simulink model "FOC_LSM"  (R2026a)
settings: Solver=VariableStepAuto  StopTime=5  MaxStep=0.001
values from neighbouring files (symbols this model uses):
  airgap_vec = 14.5:1:16.5    [CargarDatosModeloLSM.m]
  force_drag_vec = []    [CargarDatosModeloLSM.m]
  hems_n = 4    [CargarDatosModeloLSM.m]
  kd = 0.0518    [CargarDatosModeloLSM.m]
  mass = 250    [CargarDatosModeloLSM.m]
  max_current = 100    [CargarDatosModeloLSM.m]
  max_voltage = 300    [CargarDatosModeloLSM.m]
  real_airgap = 14.5    [CargarDatosModeloLSM.m]
  speed_drag_vec = 0:5:60    [CargarDatosModeloLSM.m]
undefined symbols (not defined in the file or in its folder): angulos, frac_polar, fuerza, magnitude, Resistencia
libraries: slpidlib x3
settings Model: Creator=USUARIO  LastModifiedBy=osganig
settings SolverCC: InitialStep=0.000001
settings SimscapeCC: SimscapeNominalValues="[{\"value\":\"1\",\"unit\":\"A\"},{\"value\":\"1\",\"unit\":\"bar\"},{\"value\":\"1\",\"unit\":\"cm^2\"},{\"value\":\"1\",\"unit\":\"cm^3/s\"},{\"value\":\"1\",\"unit\":\"kJ/kg\"},{\"value\":\"1\",\"unit\":\"kW\"},{\"value\":\"1\",\"unit\":\"l\"},{\"value\":\"1\",\"unit\":\"N\"},{\"value\":\"1\",\"unit\":\"N*m\"},{\"value\":\"1\",\"unit\":\"V\"}]"  SimscapeLogType=none  SimscapeLogDataHistory=5000.0

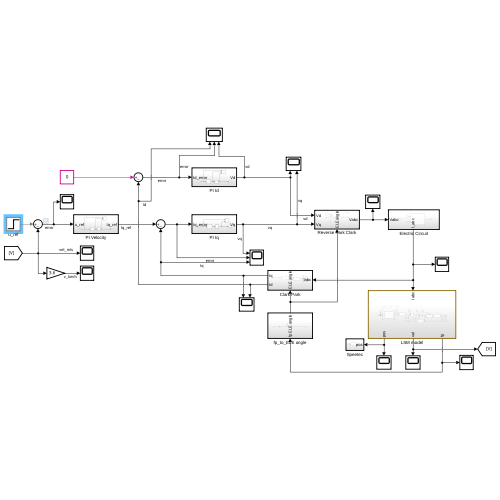
[thumbnail: Simulink's stored preview of the top-level diagram]
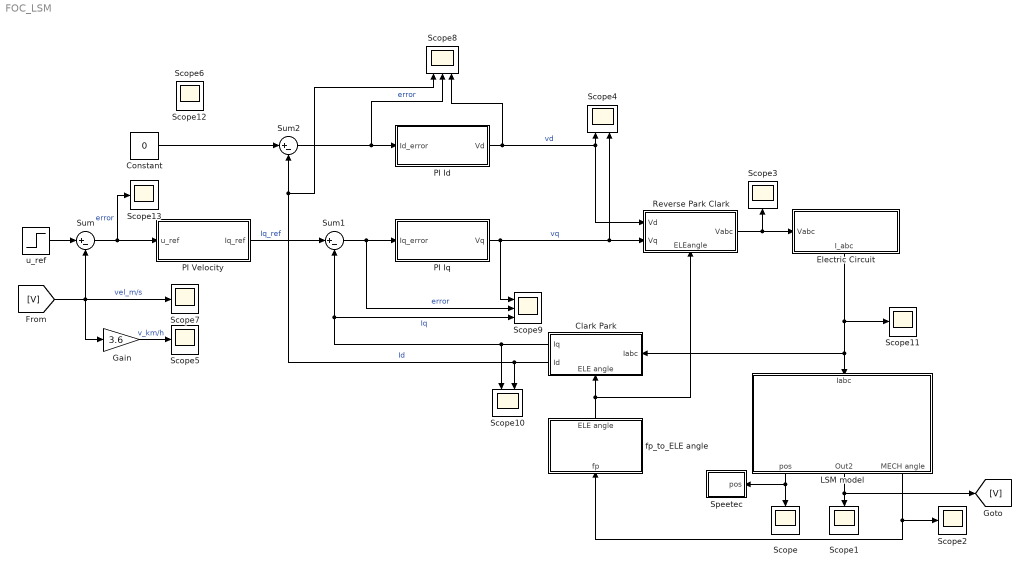
== system FOC_LSM ==
  Clark Park : Subsystem
      settings: PortSchema="{\"entries\":[{\"content\":{\"sides\":[{\"content\":{\"connectorIds\":[\"Out1\",\"Out2\"]},\"type\":\"ConnectorPlacement.EquallySpacedRectSide\",\"uuid\":\"b73a0972-bf68-45ae-9239-d3343df02446\"},{\"content\":{\"connectorIds\":[\"In2\"],\"side\":\"RIGHT\"},\"type\":\"ConnectorPlacement.EquallySpacedRectSide\",\"uuid\":\"fec89271-c2ef-4885-992a-4c0db260d6e2\"},{\"content\":{\"side\":\"TOP\"},\"type\":\"ConnectorPlacement.EquallySpacedRectSide\",\"uuid\":\"51dbb3d3-34a9-43d7-9c98-9fa2f2011719\"},{\"content\":{\"connectorIds\":[\"In1\"],\"side\":\"BOTTOM\"},\"type\":\"ConnectorPlacement.EquallySpacedRectSide\",\"uuid\":\"eab6f42e-44ed-4b27-921c-43f03788cacc\"}]},\"type\":\"ConnectorPlacement.EquallySpacedConnector\",\"uuid\":\"a64495c7-a005-4dee-b109-5230f9247adc\"}],\"packageUris\":[\"http://schema.mathworks.com/mf0/Connector/R2020b\"],\"version\":\"1.0\"}"
  Constant : Constant  Value=0
  Electric Circuit : Subsystem
      settings: PortSchema="{\"entries\":[{\"content\":{\"sides\":[{\"content\":{\"connectorIds\":[\"In1\"]},\"type\":\"ConnectorPlacement.EquallySpacedRectSide\",\"uuid\":\"3f81a6db-fb69-453a-a09a-736cf4e6fbdf\"},{\"content\":{\"side\":\"RIGHT\"},\"type\":\"ConnectorPlacement.EquallySpacedRectSide\",\"uuid\":\"28f19065-0fce-4caf-9d5e-808d35e6acc4\"},{\"content\":{\"side\":\"TOP\"},\"type\":\"ConnectorPlacement.EquallySpacedRectSide\",\"uuid\":\"0f0f3d94-64b2-4ad8-85c5-3a76de2037a2\"},{\"content\":{\"connectorIds\":[\"Out1\"],\"side\":\"BOTTOM\"},\"type\":\"ConnectorPlacement.EquallySpacedRectSide\",\"uuid\":\"1e961944-9c4a-4342-972a-1097eb822071\"}]},\"type\":\"ConnectorPlacement.EquallySpacedConnector\",\"uuid\":\"ca84a14e-6f4b-4b2e-8a9f-b6683e76143b\"}],\"packageUris\":[\"http://schema.mathworks.com/mf0/Connector/R2020b\"],\"version\":\"1.0\"}"
  Gain : Gain  Gain=3.6
  LSM model : Subsystem
      settings: PortSchema="{\"entries\":[{\"content\":{\"sides\":[{\"content\":{},\"type\":\"ConnectorPlacement.EquallySpacedRectSide\",\"uuid\":\"cac53d69-c428-44dc-bdf5-c688872b0596\"},{\"content\":{\"side\":\"RIGHT\"},\"type\":\"ConnectorPlacement.EquallySpacedRectSide\",\"uuid\":\"eab58244-5d35-448a-9540-885c93543b87\"},{\"content\":{\"connectorIds\":[\"In1\"],\"side\":\"TOP\"},\"type\":\"ConnectorPlacement.EquallySpacedRectSide\",\"uuid\":\"c64ce138-6960-4dd5-9e90-e1ffecc69b70\"},{\"content\":{\"connectorIds\":[\"Out1\",\"Out2\",\"Out3\"],\"side\":\"BOTTOM\"},\"type\":\"ConnectorPlacement.EquallySpacedRectSide\",\"uuid\":\"eda83129-b662-4da7-9603-68b1882420cc\"}]},\"type\":\"ConnectorPlacement.EquallySpacedConnector\",\"uuid\":\"82b650b8-86c6-4f03-ba07-634d14e4b94d\"}],\"packageUris\":[\"http://schema.mathworks.com/mf0/Connector/R2020b\"],\"version\":\"1.0\"}"
  PI Id : Subsystem
  PI Iq : Subsystem
  PI Velocity : Subsystem
  Reverse Park Clark : Subsystem
      settings: PortSchema="{\"entries\":[{\"content\":{\"sides\":[{\"content\":{\"connectorIds\":[\"In1\",\"In2\"]},\"type\":\"ConnectorPlacement.EquallySpacedRectSide\",\"uuid\":\"bb4b1d20-48ba-4b2f-b253-a250226ab501\"},{\"content\":{\"connectorIds\":[\"Out1\"],\"side\":\"RIGHT\"},\"type\":\"ConnectorPlacement.EquallySpacedRectSide\",\"uuid\":\"4768cfae-b67e-4820-9de3-2f5fe637e53a\"},{\"content\":{\"side\":\"TOP\"},\"type\":\"ConnectorPlacement.EquallySpacedRectSide\",\"uuid\":\"af639b0a-05db-45f8-bbbc-8f88455894ca\"},{\"content\":{\"connectorIds\":[\"In3\"],\"side\":\"BOTTOM\"},\"type\":\"ConnectorPlacement.EquallySpacedRectSide\",\"uuid\":\"149993ad-8fc7-43c9-baef-e4c40b0fb2ea\"}]},\"type\":\"ConnectorPlacement.EquallySpacedConnector\",\"uuid\":\"6dc62ad4-a38d-4494-a0f6-179f186f788d\"}],\"packageUris\":[\"http://schema.mathworks.com/mf0/Connector/R2020b\"],\"version\":\"1.0\"}"
  Scope{,1..3,5..7,11..13} (10 alike) : Scope
      Scope settings: ActiveDisplayYMinimum=-44.742643524791177  ActiveDisplayYMaximum=63.649983628393485
      Scope1 settings: ActiveDisplayYMinimum=-1  ActiveDisplayYMaximum=1  DataLoggingVariableName=ScopeData2
      Scope11 settings: ActiveDisplayYMinimum=-239.32432239172496  ActiveDisplayYMaximum=188.83608076645984  DataLoggingVariableName=ScopeData8
      Scope13 settings: ActiveDisplayYMinimum=-4.7371182514863284  ActiveDisplayYMaximum=8.95741762391783  DataLoggingVariableName=ScopeData26
      Scope2 settings: ActiveDisplayYMinimum=-0.25  ActiveDisplayYMaximum=2.25  DataLoggingVariableName=ScopeData3
      Scope3 settings: ActiveDisplayYMinimum=-282.3019987095613  ActiveDisplayYMaximum=236.76374680543654  DataLoggingVariableName=ScopeData7
      Scope5 settings: ActiveDisplayYMinimum=-77.099854779742387  ActiveDisplayYMaximum=22.66504143319689  DataLoggingVariableName=ScopeData22
      Scope7 settings: ActiveDisplayYMinimum=4.6850634488954057  ActiveDisplayYMaximum=8.1784524143386932  DataLoggingVariableName=ScopeData17
      Scope12 settings: DataLoggingVariableName=ScopeData24
      Scope6 settings: ActiveDisplayYMinimum=-26.658365067541684  ActiveDisplayYMaximum=23.617816668325265  DataLoggingVariableName=ScopeData23
  Scope10 : Scope  NumInputPorts=2
      settings: ActiveDisplayYMinimum=-159.849934056899  ActiveDisplayYMaximum=156.59274633785697  DataLoggingVariableName=ScopeData21
  Scope4 : Scope  NumInputPorts=2
      settings: ActiveDisplayYMinimum=-644.81411467829275  ActiveDisplayYMaximum=391.29333465512445  DataLoggingVariableName=ScopeData9
  Scope8 : Scope  NumInputPorts=3
      settings: ActiveDisplayYMinimum=-641.93741582792154  ActiveDisplayYMaximum=154.89056521574875  DataLoggingVariableName=ScopeData18
  Scope9 : Scope  NumInputPorts=3
      settings: ActiveDisplayYMinimum=-2.3010895783885954  ActiveDisplayYMaximum=2.3440027579560128  DataLoggingVariableName=ScopeData19
  Speetec : Subsystem
  Sum : Sum  Inputs=|+-
  Sum1 : Sum  Inputs=|+-
  Sum2 : Sum  Inputs=|+-
  fp_to_ELE angle : Subsystem
      settings: PortSchema="{\"entries\":[{\"content\":{\"sides\":[{\"content\":{},\"type\":\"ConnectorPlacement.EquallySpacedRectSide\",\"uuid\":\"b73a0972-bf68-45ae-9239-d3343df02446\"},{\"content\":{\"side\":\"RIGHT\"},\"type\":\"ConnectorPlacement.EquallySpacedRectSide\",\"uuid\":\"fec89271-c2ef-4885-992a-4c0db260d6e2\"},{\"content\":{\"connectorIds\":[\"Out1\"],\"side\":\"TOP\"},\"type\":\"ConnectorPlacement.EquallySpacedRectSide\",\"uuid\":\"51dbb3d3-34a9-43d7-9c98-9fa2f2011719\"},{\"content\":{\"connectorIds\":[\"In1\"],\"side\":\"BOTTOM\"},\"type\":\"ConnectorPlacement.EquallySpacedRectSide\",\"uuid\":\"4816d69c-9e54-4057-b439-390caef350ee\"}]},\"type\":\"ConnectorPlacement.EquallySpacedConnector\",\"uuid\":\"a64495c7-a005-4dee-b109-5230f9247adc\"}],\"packageUris\":[\"http://schema.mathworks.com/mf0/Connector/R2020b\"],\"version\":\"1.0\"}"
  u_ref : Step  FinalValue=speed_reference_ms  SampleTime=0
  wires:
  Constant/1 -> Sum2/1
  LSM model/3(MECH angle) -> fp_to_ELE angle/1(fp), Scope2/1
  Clark Park/2(Id) -> Scope10/2, Scope8/1, Sum2/2  "Id"
  fp_to_ELE angle/1(ELE angle) -> Reverse Park Clark/3(ELEangle), Clark Park/1(ELE angle)
  Clark Park/1(Iq) -> Scope10/1, Scope9/3, Sum1/2  "Iq"
  Electric Circuit/1(I_abc) -> LSM model/1(Iabc), Clark Park/2(Iabc), Scope11/1
  u_ref/1 -> Sum/1
  Sum1/1 -> PI Iq/1(Iq_error), Scope9/2  "error"
  LSM model/1(pos) -> Scope/1, Speetec/1(pos)
  LSM model/2(Out2) -> Scope1/1, [V]
  PI Id/1(Vd) -> Scope8/3, Reverse Park Clark/1(Vd), Scope4/1  "vd"
  [V] -> Scope7/1, Gain/1, Sum/2  "vel_m/s"
  Sum/1 -> Scope13/1, PI Velocity/1(u_ref)  "error"
  Sum2/1 -> PI Id/1(Id_error), Scope8/2  "error"
  PI Iq/1(Vq) -> Reverse Park Clark/2(Vq), Scope4/2, Scope9/1  "vq"
  Reverse Park Clark/1(Vabc) -> Electric Circuit/1(Vabc), Scope3/1
  PI Velocity/1(Iq_ref) -> Sum1/1  "Iq_ref"
  Gain/1 -> Scope5/1  "v_km/h"

== system FOC_LSM/Clark Park ==
  ELE angle : Inport
  Iabc : Inport  Port=2
  Clarke Transform : MATLAB Function  TreatAsAtomicUnit=on
  Clarke to Park Angle Transform : MATLAB Function  TreatAsAtomicUnit=on
  Demux : Demux  Outputs=3
  Terminator : Terminator
  Iq : Outport
  Id : Outport  Port=2
  wires:
  Iabc/1 -> Clarke Transform/1(abc)
  ELE angle/1 -> Clarke to Park Angle Transform/2(ELE_angle)
  Clarke to Park Angle Transform/1(dq0) -> Demux/1
  Demux/1 -> Id/1
  Demux/2 -> Iq/1
  Demux/3 -> Terminator/1
  Clarke Transform/1(AlphaBeta0) -> Clarke to Park Angle Transform/1(AlphaBeta0)

== system FOC_LSM/Electric Circuit ==
  Vabc : Inport
  Constant : Constant  Value=0.01
  Equivalente eléctrico : Subsystem
  I_abc : Outport
  wires:
  Equivalente eléctrico/1(I UVW) -> I_abc/1
  [V_abc] -> Equivalente eléctrico/2(Voltaje)
  Constant/1 -> Equivalente eléctrico/1(Inductancia)
  Vabc/1 -> [V_abc]

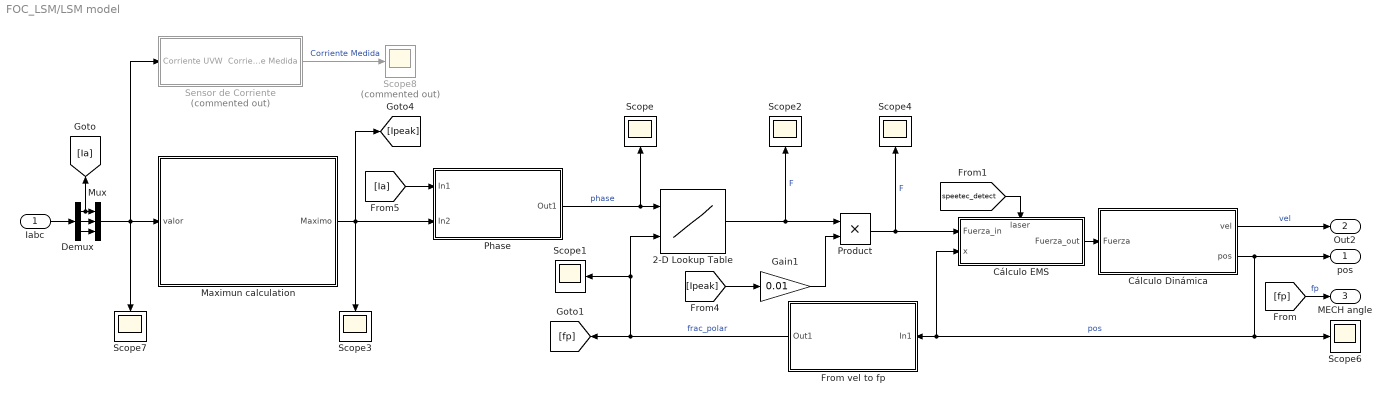
== system FOC_LSM/LSM model ==
  Iabc : Inport
  2-D Lookup Table : Lookup_n-D  BreakpointsForDimension1=angulos  BreakpointsForDimension2=frac_polar  Table=fuerza  InternalRulePriority=Speed  RndMeth=Simplest
      settings: InputPortMap=u0,u1
  Cálculo Dinámica : Subsystem
  Cálculo EMS : Subsystem
      settings: PortSchema="{\"entries\":[{\"content\":{\"sides\":[{\"content\":{\"connectorIds\":[\"In1\",\"In2\"]},\"type\":\"ConnectorPlacement.EquallySpacedRectSide\",\"uuid\":\"594e4846-1a49-4859-b5fd-6d3523a2d917\"},{\"content\":{\"connectorIds\":[\"Out1\"],\"side\":\"RIGHT\"},\"type\":\"ConnectorPlacement.EquallySpacedRectSide\",\"uuid\":\"ea9ee920-6e59-403e-8f5a-e9dd28db2a53\"},{\"content\":{\"connectorIds\":[\"In3\"],\"side\":\"TOP\"},\"type\":\"ConnectorPlacement.EquallySpacedRectSide\",\"uuid\":\"15b2c308-55de-42ee-8b35-dfe14c52728c\"}]},\"type\":\"ConnectorPlacement.EquallySpacedConnector\",\"uuid\":\"9cb68d56-cad5-4175-b4c3-a37da794ea4d\"}],\"packageUris\":[\"http://schema.mathworks.com/mf0/Connector/R2020b\"],\"version\":\"1.0\"}"
  Demux : Demux  Outputs=3
  From vel to fp : Subsystem
  Gain1 : Gain  Gain=0.01
  Maximun calculation : Subsystem
  Mux : Mux  Inputs=3
  Phase : Subsystem
  Product : Product
  Scope{,1..4,6..7} (7 alike) : Scope
      Scope settings: ActiveDisplayYMinimum=-2.74889  ActiveDisplayYMaximum=9.03208  DataLoggingVariableName=ScopeData5
      Scope1 settings: ActiveDisplayYMinimum=-0.24999  ActiveDisplayYMaximum=2.24993  DataLoggingVariableName=ScopeData6
      Scope2 settings: ActiveDisplayYMinimum=-562.86836  ActiveDisplayYMaximum=703.0646  DataLoggingVariableName=ScopeData7
      Scope3 settings: ActiveDisplayYMinimum=-12.44358  ActiveDisplayYMaximum=111.99326  DataLoggingVariableName=ScopeData8
      Scope4 settings: ActiveDisplayYMinimum=-66.01663  ActiveDisplayYMaximum=594.14423  DataLoggingVariableName=ScopeData14
      Scope6 settings: ActiveDisplayYMinimum=-3.04039  ActiveDisplayYMaximum=27.3635  DataLoggingVariableName=ScopeData11
      Scope7 settings: ActiveDisplayYMinimum=-124.44767  ActiveDisplayYMaximum=124.44785  DataLoggingVariableName=ScopeData9
  Scope8 : Scope  Commented=on
      settings: ActiveDisplayYMinimum=-99.89011  ActiveDisplayYMaximum=99.74359  DataLoggingVariableName=ScopeData10
  Sensor de Corriente : Subsystem  Commented=on
  pos : Outport
  Out2 : Outport  Port=2
  MECH angle : Outport  Port=3
  wires:
  Gain1/1 -> Product/2
  Maximun calculation/1(Maximo) -> Scope3/1, Phase/2(In2), [Ipeak]
  Phase/1(Out1) -> 2-D Lookup Table/1, Scope/1  "phase"
  2-D Lookup Table/1 -> Product/1, Scope2/1  "F"
  From vel to fp/1(Out1) -> 2-D Lookup Table/2, Scope1/1, [fp]  "frac_polar"
  Demux/1 -> [Ia], Mux/1
  Demux/2 -> Mux/2
  Demux/3 -> Mux/3
  Mux/1 -> Scope7/1, Sensor de Corriente/1(Corriente UVW), Maximun calculation/1(valor)
  [Ipeak] -> Gain1/1
  [Ia] -> Phase/1(In1)
  Sensor de Corriente/1(Corriente Medida) -> Scope8/1  "Corriente Medida"
  Iabc/1 -> Demux/1
  [fp] -> MECH angle/1  "fp"
  Product/1 -> Scope4/1, Cálculo EMS/1(Fuerza_in)  "F"
  [speetec_detect] -> Cálculo EMS/3(laser)
  Cálculo EMS/1(Fuerza_out) -> Cálculo Dinámica/1(Fuerza)
  Cálculo Dinámica/2(pos) -> pos/1, Scope6/1, Cálculo EMS/2(x), From vel to fp/1(In1)  "pos"
  Cálculo Dinámica/1(vel) -> Out2/1  "vel"

== system FOC_LSM/PI Id ==
  Id_error : Inport
  PID Controller : slpidlib/PID Controller  Controller=PI  Form=Parallel  TimeDomain=Continuous-time  UseExternalTs=off  SampleTime=-1  IntegratorMethod=Forward Euler  FilterMethod=Forward Euler  ControllerParametersSource=internal  P=200  I=200  UseKiTs=off  D=0  UseExternalDerivativeSource=off  N=100  UseFilter=on  TunerSelectOption=Transfer Function Based (PID Tuner App)  InitialConditionSource=internal  InitialConditionForIntegrator=0  InitialConditionForFilter=0  DifferentiatorICPrevScaledInput=0  ExternalReset=none  TrackingMode=off  Kt=1  LimitOutput=off  SatLimitsSource=internal  UpperSaturationLimit=inf  LowerSaturationLimit=-inf  LinearizeAsGain=on  AntiWindupMode=none  Kb=1  LimitIntegrator=off  UpperIntegratorSaturationLimit=inf  LowerIntegratorSaturationLimit=-inf  POutMin=[]  POutMax=[]  IOutMin=[]  IOutMax=[]  DOutMin=[]  DOutMax=[]  NOutMin=[]  NOutMax=[]  SumOutMin=[]  SumOutMax=[]  SaturationOutMin=[]  SaturationOutMax=[]  PParamMin=[]  PParamMax=[]  IParamMin=[]  IParamMax=[]  DParamMin=[]  DParamMax=[]  NParamMin=[]  NParamMax=[]  KbParamMin=[]  KbParamMax=[]  KtParamMin=[]  KtParamMax=[]  KbOutMin=[]  KbOutMax=[]  KtOutMin=[]  KtOutMax=[]  IntegratorOutMin=[]  IntegratorOutMax=[]  FilterOutMin=[]  FilterOutMax=[]  SumI1OutMin=[]  SumI1OutMax=[]  SumI2OutMin=[]  SumI2OutMax=[]  SumI3OutMin=[]  SumI3OutMax=[]  SumI4OutMin=[]  SumI4OutMax=[]  SumDOutMin=[]  SumDOutMax=[]  DifferentiatorOutMin=[]  DifferentiatorOutMax=[]  FilterDiffOutCoefMin=[]  FilterDiffOutCoefMax=[]  ReciprocalOutMin=[]  ReciprocalOutMax=[]  SumDenOutMin=[]  SumDenOutMax=[]  SumNumOutMin=[]  SumNumOutMax=[]  DivideOutMin=[]  DivideOutMax=[]  UdiffTsProdOutMin=[]  UdiffTsProdOutMax=[]  NTsProdOutMin=[]  NTsProdOutMax=[]  UintegralTsProdOutMin=[]  UintegralTsProdOutMax=[]  UngainTsProdOutMin=[]  UngainTsProdOutMax=[]  ClampingZeroOutDataTypeStr=Inherit: Inherit via back propagation  ClampingZeroOutMin=[]  ClampingZeroOutMax=[]  FilterDenConstantOutDataTypeStr=Inherit: Inherit via back propagation  FilterDenConstantOutMin=[]  FilterDenConstantOutMax=[]  PCopyOutDataTypeStr=Inherit: Inherit via back propagation  PCopyOutMin=[]  PCopyOutMax=[]  NCopyOutDataTypeStr=Inherit: Inherit via back propagation  NCopyOutMin=[]  NCopyOutMax=[]  IntegratorContinuousStateAttributes=''  IntegratorStateMustResolveToSignalObject=off  IntegratorRTWStateStorageClass=Auto  FilterContinuousStateAttributes=''  FilterStateMustResolveToSignalObject=off  FilterRTWStateStorageClass=Auto  ParallelPVariant=InternalParameters  IdealPVariant=Disabled  IVariant=InternalParameters  DVariant=Disabled  IntegratorVariant=Continuous  SatVariant=Disabled  AWVariant=Passthrough  PCopyVariant=Disabled  TRVariant=Disabled  FdbkBlocksVariant=Forward  IdealPFdbkVariant=Disabled  SatFdbkVariant=Disabled  DerivativeFilterVariant=Disabled  NVariant=Disabled  NCopyVariant=Disabled_SignalSpec  FilterICVariant=Disabled  IntegratorICVariant=InternalICs  ExternalResetVariant=Disabled  TRSumVariant=Passthrough  SumFdbkVariant=Disabled  SumVariant=Sum_PI  TsampFilterVariant=InternalTs  TsampNgainVariant=Passthrough  TsampIntegralVariant=Disabled_SignalSpec  ExternalSaturationOutDataTypeStr=Inherit: Same as second input  DerivativeSourceVariant=Disabled  PreIntVariant=InternalPreInt
  Saturation3 : Saturate  UpperLimit=max_voltage  LowerLimit=-max_voltage
  Scope : Scope  NumInputPorts=3
      settings: ActiveDisplayYMinimum=-3.33517  ActiveDisplayYMaximum=0.987  DataLoggingVariableName=ScopeData20
  Vd : Outport
  wires:
  Id_error/1 -> PID Controller/1, Scope/1
  Saturation3/1 -> Scope/3, Vd/1
  PID Controller/1 -> Scope/2, Saturation3/1  "vd"

== system FOC_LSM/PI Iq ==
  Iq_error : Inport
  PID Controller1 : slpidlib/PID Controller  Controller=PI  Form=Parallel  TimeDomain=Continuous-time  UseExternalTs=off  SampleTime=-1  IntegratorMethod=Forward Euler  FilterMethod=Forward Euler  ControllerParametersSource=internal  P=50  I=50  UseKiTs=off  D=0  UseExternalDerivativeSource=off  N=100  UseFilter=on  TunerSelectOption=Transfer Function Based (PID Tuner App)  InitialConditionSource=internal  InitialConditionForIntegrator=0  InitialConditionForFilter=0  DifferentiatorICPrevScaledInput=0  ExternalReset=none  TrackingMode=off  Kt=1  LimitOutput=off  SatLimitsSource=internal  UpperSaturationLimit=inf  LowerSaturationLimit=-inf  LinearizeAsGain=on  AntiWindupMode=none  Kb=1  LimitIntegrator=off  UpperIntegratorSaturationLimit=inf  LowerIntegratorSaturationLimit=-inf  POutMin=[]  POutMax=[]  IOutMin=[]  IOutMax=[]  DOutMin=[]  DOutMax=[]  NOutMin=[]  NOutMax=[]  SumOutMin=[]  SumOutMax=[]  SaturationOutMin=[]  SaturationOutMax=[]  PParamMin=[]  PParamMax=[]  IParamMin=[]  IParamMax=[]  DParamMin=[]  DParamMax=[]  NParamMin=[]  NParamMax=[]  KbParamMin=[]  KbParamMax=[]  KtParamMin=[]  KtParamMax=[]  KbOutMin=[]  KbOutMax=[]  KtOutMin=[]  KtOutMax=[]  IntegratorOutMin=[]  IntegratorOutMax=[]  FilterOutMin=[]  FilterOutMax=[]  SumI1OutMin=[]  SumI1OutMax=[]  SumI2OutMin=[]  SumI2OutMax=[]  SumI3OutMin=[]  SumI3OutMax=[]  SumI4OutMin=[]  SumI4OutMax=[]  SumDOutMin=[]  SumDOutMax=[]  DifferentiatorOutMin=[]  DifferentiatorOutMax=[]  FilterDiffOutCoefMin=[]  FilterDiffOutCoefMax=[]  ReciprocalOutMin=[]  ReciprocalOutMax=[]  SumDenOutMin=[]  SumDenOutMax=[]  SumNumOutMin=[]  SumNumOutMax=[]  DivideOutMin=[]  DivideOutMax=[]  UdiffTsProdOutMin=[]  UdiffTsProdOutMax=[]  NTsProdOutMin=[]  NTsProdOutMax=[]  UintegralTsProdOutMin=[]  UintegralTsProdOutMax=[]  UngainTsProdOutMin=[]  UngainTsProdOutMax=[]  ClampingZeroOutDataTypeStr=Inherit: Inherit via back propagation  ClampingZeroOutMin=[]  ClampingZeroOutMax=[]  FilterDenConstantOutDataTypeStr=Inherit: Inherit via back propagation  FilterDenConstantOutMin=[]  FilterDenConstantOutMax=[]  PCopyOutDataTypeStr=Inherit: Inherit via back propagation  PCopyOutMin=[]  PCopyOutMax=[]  NCopyOutDataTypeStr=Inherit: Inherit via back propagation  NCopyOutMin=[]  NCopyOutMax=[]  IntegratorContinuousStateAttributes=''  IntegratorStateMustResolveToSignalObject=off  IntegratorRTWStateStorageClass=Auto  FilterContinuousStateAttributes=''  FilterStateMustResolveToSignalObject=off  FilterRTWStateStorageClass=Auto  ParallelPVariant=InternalParameters  IdealPVariant=Disabled  IVariant=InternalParameters  DVariant=Disabled  IntegratorVariant=Continuous  SatVariant=Disabled  AWVariant=Passthrough  PCopyVariant=Disabled  TRVariant=Disabled  FdbkBlocksVariant=Forward  IdealPFdbkVariant=Disabled  SatFdbkVariant=Disabled  DerivativeFilterVariant=Disabled  NVariant=Disabled  NCopyVariant=Disabled_SignalSpec  FilterICVariant=Disabled  IntegratorICVariant=InternalICs  ExternalResetVariant=Disabled  TRSumVariant=Passthrough  SumFdbkVariant=Disabled  SumVariant=Sum_PI  TsampFilterVariant=InternalTs  TsampNgainVariant=Passthrough  TsampIntegralVariant=Disabled_SignalSpec  ExternalSaturationOutDataTypeStr=Inherit: Same as second input  DerivativeSourceVariant=Disabled  PreIntVariant=InternalPreInt
  Saturation : Saturate  UpperLimit=max_voltage  LowerLimit=-max_voltage
  Scope : Scope  NumInputPorts=2
      settings: ActiveDisplayYMinimum=-70.69088  ActiveDisplayYMaximum=255.57471  DataLoggingVariableName=ScopeData22
  Vq : Outport
  wires:
  Iq_error/1 -> Scope/1, PID Controller1/1
  Saturation/1 -> Scope/2, Vq/1
  PID Controller1/1 -> Saturation/1

== system FOC_LSM/PI Velocity ==
  u_ref : Inport
  PID Controller : slpidlib/PID Controller  Controller=PI  Form=Parallel  TimeDomain=Continuous-time  UseExternalTs=off  SampleTime=-1  IntegratorMethod=Forward Euler  FilterMethod=Forward Euler  ControllerParametersSource=internal  P=6  I=15  UseKiTs=off  D=0  UseExternalDerivativeSource=off  N=100  UseFilter=on  TunerSelectOption=Transfer Function Based (PID Tuner App)  InitialConditionSource=internal  InitialConditionForIntegrator=0  InitialConditionForFilter=0  DifferentiatorICPrevScaledInput=0  ExternalReset=none  TrackingMode=off  Kt=1  LimitOutput=off  SatLimitsSource=internal  UpperSaturationLimit=inf  LowerSaturationLimit=-inf  LinearizeAsGain=on  AntiWindupMode=none  Kb=1  LimitIntegrator=off  UpperIntegratorSaturationLimit=inf  LowerIntegratorSaturationLimit=-inf  POutMin=[]  POutMax=[]  IOutMin=[]  IOutMax=[]  DOutMin=[]  DOutMax=[]  NOutMin=[]  NOutMax=[]  SumOutMin=[]  SumOutMax=[]  SaturationOutMin=[]  SaturationOutMax=[]  PParamMin=[]  PParamMax=[]  IParamMin=[]  IParamMax=[]  DParamMin=[]  DParamMax=[]  NParamMin=[]  NParamMax=[]  KbParamMin=[]  KbParamMax=[]  KtParamMin=[]  KtParamMax=[]  KbOutMin=[]  KbOutMax=[]  KtOutMin=[]  KtOutMax=[]  IntegratorOutMin=[]  IntegratorOutMax=[]  FilterOutMin=[]  FilterOutMax=[]  SumI1OutMin=[]  SumI1OutMax=[]  SumI2OutMin=[]  SumI2OutMax=[]  SumI3OutMin=[]  SumI3OutMax=[]  SumI4OutMin=[]  SumI4OutMax=[]  SumDOutMin=[]  SumDOutMax=[]  DifferentiatorOutMin=[]  DifferentiatorOutMax=[]  FilterDiffOutCoefMin=[]  FilterDiffOutCoefMax=[]  ReciprocalOutMin=[]  ReciprocalOutMax=[]  SumDenOutMin=[]  SumDenOutMax=[]  SumNumOutMin=[]  SumNumOutMax=[]  DivideOutMin=[]  DivideOutMax=[]  UdiffTsProdOutMin=[]  UdiffTsProdOutMax=[]  NTsProdOutMin=[]  NTsProdOutMax=[]  UintegralTsProdOutMin=[]  UintegralTsProdOutMax=[]  UngainTsProdOutMin=[]  UngainTsProdOutMax=[]  ClampingZeroOutDataTypeStr=Inherit: Inherit via back propagation  ClampingZeroOutMin=[]  ClampingZeroOutMax=[]  FilterDenConstantOutDataTypeStr=Inherit: Inherit via back propagation  FilterDenConstantOutMin=[]  FilterDenConstantOutMax=[]  PCopyOutDataTypeStr=Inherit: Inherit via back propagation  PCopyOutMin=[]  PCopyOutMax=[]  NCopyOutDataTypeStr=Inherit: Inherit via back propagation  NCopyOutMin=[]  NCopyOutMax=[]  IntegratorContinuousStateAttributes=''  IntegratorStateMustResolveToSignalObject=off  IntegratorRTWStateStorageClass=Auto  FilterContinuousStateAttributes=''  FilterStateMustResolveToSignalObject=off  FilterRTWStateStorageClass=Auto  ParallelPVariant=InternalParameters  IdealPVariant=Disabled  IVariant=InternalParameters  DVariant=Disabled  IntegratorVariant=Continuous  SatVariant=Disabled  AWVariant=Passthrough  PCopyVariant=Disabled  TRVariant=Disabled  FdbkBlocksVariant=Forward  IdealPFdbkVariant=Disabled  SatFdbkVariant=Disabled  DerivativeFilterVariant=Disabled  NVariant=Disabled  NCopyVariant=Disabled_SignalSpec  FilterICVariant=Disabled  IntegratorICVariant=InternalICs  ExternalResetVariant=Disabled  TRSumVariant=Passthrough  SumFdbkVariant=Disabled  SumVariant=Sum_PI  TsampFilterVariant=InternalTs  TsampNgainVariant=Passthrough  TsampIntegralVariant=Disabled_SignalSpec  ExternalSaturationOutDataTypeStr=Inherit: Same as second input  DerivativeSourceVariant=Disabled  PreIntVariant=InternalPreInt
  Saturation2 : Saturate  UpperLimit=max_current  LowerLimit=0
  Scope : Scope  NumInputPorts=3
      settings: ActiveDisplayYMinimum=-316.67869889181191  ActiveDisplayYMaximum=367.95314738582192  DataLoggingVariableName=ScopeData15
  Iq_ref : Outport
  wires:
  u_ref/1 -> PID Controller/1, Scope/1
  PID Controller/1 -> Scope/2, Saturation2/1
  Saturation2/1 -> Scope/3, Iq_ref/1  "Iq_ref"

== system FOC_LSM/Reverse Park Clark ==
  Vd : Inport
  Vq : Inport  Port=2
  ELEangle : Inport  Port=3
  Constant : Constant  Value=0
  Inverse Park Transform : MATLAB Function  TreatAsAtomicUnit=on
  Mux : Mux  Inputs=3
  Scope : Scope
      settings: ActiveDisplayYMinimum=-353.32237  ActiveDisplayYMaximum=282.12386
  Scope1 : Scope
      settings: ActiveDisplayYMinimum=-1.5976804907047262  ActiveDisplayYMaximum=7.4603893364098015  DataLoggingVariableName=ScopeData3
  Vabc : Outport
  wires:
  Vd/1 -> Mux/1
  Vq/1 -> Mux/2
  Constant/1 -> Mux/3
  Mux/1 -> Inverse Park Transform/1(dq0)
  ELEangle/1 -> Scope1/1, Inverse Park Transform/2(ELE_angle)
  Inverse Park Transform/1(abc) -> Scope/1, Vabc/1

== system FOC_LSM/Speetec ==
  pos : Inport
  Speetec Detection : MATLAB Function  TreatAsAtomicUnit=on
  tag scope: speetec_detect=global
  wires:
  pos/1 -> Speetec Detection/1(pos)
  Speetec Detection/1(speetec_detect) -> [speetec_detect]

== system FOC_LSM/fp_to_ELE angle ==
  fp : Inport
  Gain : Gain  Gain=pi
  Scope : Scope
      settings: ActiveDisplayYMinimum=2.6308154799609307  ActiveDisplayYMaximum=4.6536331019278112  DataLoggingVariableName=ScopeData4
  ELE angle : Outport
  wires:
  fp/1 -> Gain/1
  Gain/1 -> Scope/1, ELE angle/1

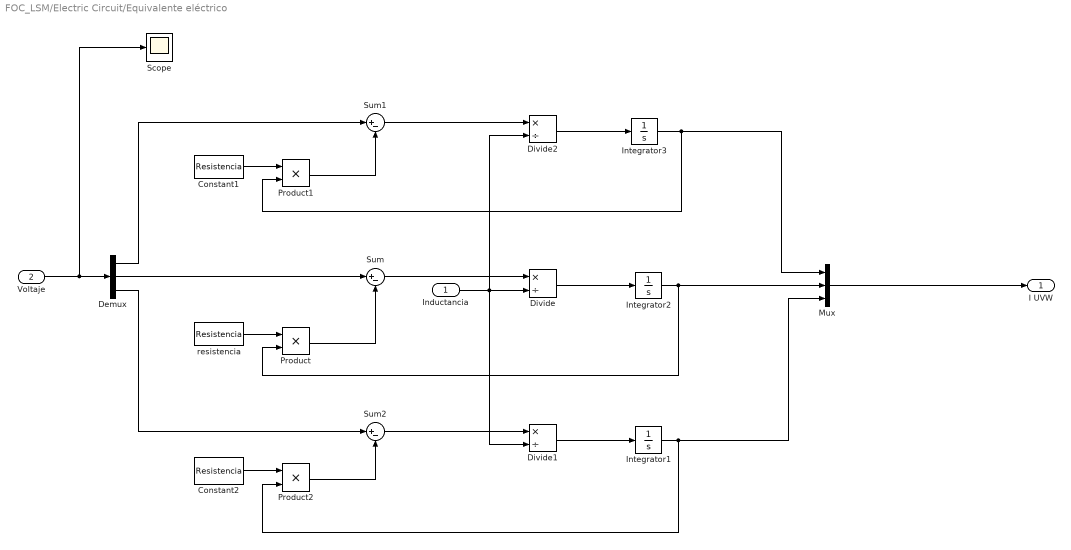
== system FOC_LSM/Electric Circuit/Equivalente eléctrico ==
  Inductancia : Inport
  Voltaje : Inport  Port=2
  Constant1 : Constant  Value=Resistencia
  Constant2 : Constant  Value=Resistencia
  Demux : Demux  Outputs=3
  Divide : Product  Inputs=*/
  Divide1 : Product  Inputs=*/
  Divide2 : Product  Inputs=*/
  Integrator1 : Integrator
  Integrator2 : Integrator
  Integrator3 : Integrator
  Mux : Mux  Inputs=3
  Product : Product
  Product1 : Product
  Product2 : Product
  Scope : Scope
      settings: ActiveDisplayYMinimum=-2.13493  ActiveDisplayYMaximum=1.34462  DataLoggingVariableName=ScopeData15
  Sum : Sum  Inputs=|+-
  Sum1 : Sum  Inputs=|+-
  Sum2 : Sum  Inputs=|+-
  resistencia : Constant  Value=Resistencia
  I UVW : Outport
  wires:
  Voltaje/1 -> Scope/1, Demux/1
  Demux/2 -> Sum/1
  Product/1 -> Sum/2
  resistencia/1 -> Product/1
  Sum/1 -> Divide/1
  Inductancia/1 -> Divide1/2, Divide2/2, Divide/2
  Product1/1 -> Sum1/2
  Sum1/1 -> Divide2/1
  Demux/1 -> Sum1/1
  Constant1/1 -> Product1/1
  Product2/1 -> Sum2/2
  Sum2/1 -> Divide1/1
  Demux/3 -> Sum2/1
  Constant2/1 -> Product2/1
  Divide2/1 -> Integrator3/1
  Integrator3/1 -> Product1/2, Mux/1
  Divide/1 -> Integrator2/1
  Divide1/1 -> Integrator1/1
  Integrator2/1 -> Product/2, Mux/2
  Integrator1/1 -> Product2/2, Mux/3
  Mux/1 -> I UVW/1

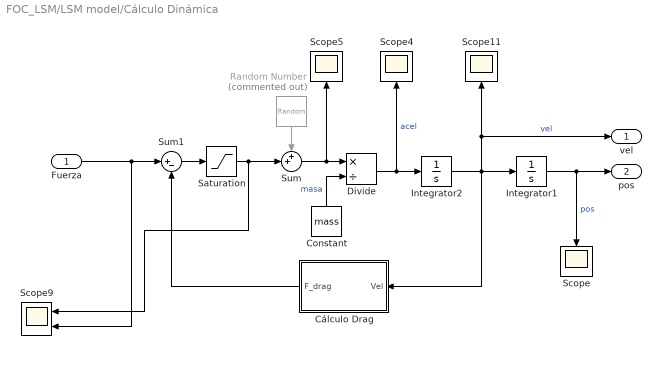
== system FOC_LSM/LSM model/Cálculo Dinámica ==
  Fuerza : Inport
  Constant : Constant  Value=mass
  Cálculo Drag : Subsystem
  Divide : Product  Inputs=*/
  Integrator1 : Integrator
  Integrator2 : Integrator  InitialCondition=1
  Random Number : RandomNumber  Commented=on  Mean=-10  SampleTime=0.1
  Saturation : Saturate  UpperLimit=inf  LowerLimit=0
  Scope{,4..5,11} (4 alike) : Scope
      Scope settings: ActiveDisplayYMinimum=-2.76412  ActiveDisplayYMaximum=24.87706  DataLoggingVariableName=ScopeData21
      Scope11 settings: ActiveDisplayYMinimum=0.26356  ActiveDisplayYMaximum=7.62797  DataLoggingVariableName=ScopeData13
      Scope4 settings: ActiveDisplayYMinimum=-1.56526  ActiveDisplayYMaximum=14.0873
      Scope5 settings: ActiveDisplayYMinimum=-391.31378  ActiveDisplayYMaximum=3521.82401  DataLoggingVariableName=ScopeData2
  Scope9 : Scope  NumInputPorts=2
      settings: ActiveDisplayYMinimum=-429.70499  ActiveDisplayYMaximum=3867.34492  DataLoggingVariableName=ScopeData2
  Sum : Sum  Inputs=++|
  Sum1 : Sum  Inputs=|+-
  vel : Outport
  pos : Outport  Port=2
  wires:
  Constant/1 -> Divide/2  "masa"
  Sum/1 -> Scope5/1, Divide/1
  Divide/1 -> Integrator2/1, Scope4/1  "acel"
  Integrator2/1 -> Cálculo Drag/1(Vel), Integrator1/1, Scope11/1, vel/1  "vel"
  Random Number/1 -> Sum/1
  Integrator1/1 -> pos/1, Scope/1  "pos"
  Fuerza/1 -> Sum1/1, Scope9/2
  Sum1/1 -> Saturation/1
  Cálculo Drag/1(F_drag) -> Sum1/2
  Saturation/1 -> Scope9/1, Sum/2

== system FOC_LSM/LSM model/Cálculo EMS ==
  note: En este bloque no está incluido el desfase del sensor
  Fuerza_in : Inport
  x : Inport  Port=2
  laser : Inport  Port=3
  Cálculo EMS : MATLAB Function  TreatAsAtomicUnit=on
  Product : Product
  Scope : Scope
      settings: ActiveDisplayYMinimum=-2.76412  ActiveDisplayYMaximum=24.87706  DataLoggingVariableName=ScopeData16
  Scope10 : Scope  NumInputPorts=2
      settings: ActiveDisplayYMinimum=-0.75  ActiveDisplayYMaximum=6.75  DataLoggingVariableName=ScopeData10
  Subsystem : Subsystem
  Fuerza_out : Outport
  wires:
  Cálculo EMS/1(numero_EMS) -> Scope10/1, Product/1
  laser/1 -> Cálculo EMS/1(laser)
  x/1 -> Subsystem/1(pos), Scope/1, Cálculo EMS/2(pos)
  Subsystem/1(Out1) -> Scope10/2  "n"
  Fuerza_in/1 -> Product/2
  Product/1 -> Fuerza_out/1

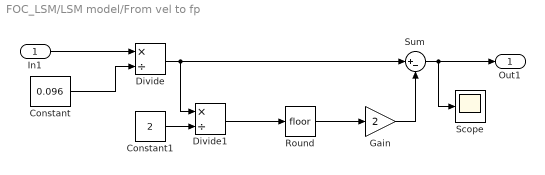
== system FOC_LSM/LSM model/From vel to fp ==
  In1 : Inport
  Constant : Constant  Value=0.096
  Constant1 : Constant  Value=2
  Divide : Product  Inputs=*/
  Divide1 : Product  Inputs=*/
  Gain : Gain  Gain=2
  Round : Rounding
  Scope : Scope
      settings: ActiveDisplayYMinimum=-0.24999  ActiveDisplayYMaximum=2.24992  DataLoggingVariableName=ScopeData3
  Sum : Sum  Inputs=|+-
  Out1 : Outport
  wires:
  In1/1 -> Divide/1
  Constant/1 -> Divide/2
  Divide/1 -> Divide1/1, Sum/1
  Divide1/1 -> Round/1
  Round/1 -> Gain/1
  Constant1/1 -> Divide1/2
  Gain/1 -> Sum/2
  Sum/1 -> Scope/1, Out1/1

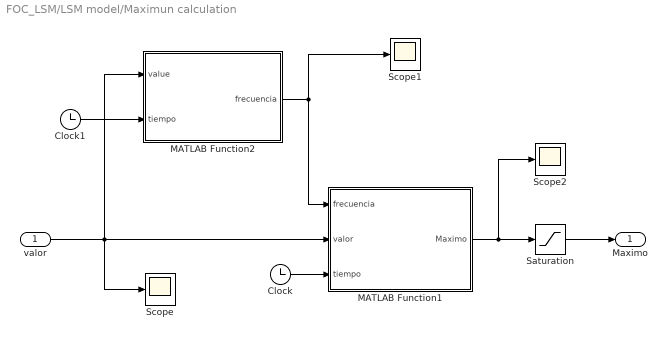
== system FOC_LSM/LSM model/Maximun calculation ==
  valor : Inport
  Clock : Clock
  Clock1 : Clock
  MATLAB Function1 : MATLAB Function  TreatAsAtomicUnit=on
  MATLAB Function2 : MATLAB Function  TreatAsAtomicUnit=on
  Saturation : Saturate  UpperLimit=inf  LowerLimit=0.0001
  Scope : Scope
      settings: ActiveDisplayYMinimum=-1.01844  ActiveDisplayYMaximum=1.01854  DataLoggingVariableName=ScopeData6
  Scope1 : Scope
      settings: ActiveDisplayYMinimum=14.240357573038054  ActiveDisplayYMaximum=27.26338877720746  DataLoggingVariableName=ScopeData7
  Scope2 : Scope
      settings: ActiveDisplayYMinimum=-1.01844  ActiveDisplayYMaximum=1.01854  DataLoggingVariableName=ScopeData25
  Maximo : Outport
  wires:
  Clock/1 -> MATLAB Function1/3(tiempo)
  MATLAB Function2/1(frecuencia) -> MATLAB Function1/1(frecuencia), Scope1/1
  Clock1/1 -> MATLAB Function2/2(tiempo)
  MATLAB Function1/1(Maximo) -> Scope2/1, Saturation/1
  Saturation/1 -> Maximo/1
  valor/1 -> Scope/1, MATLAB Function1/2(valor), MATLAB Function2/1(value)

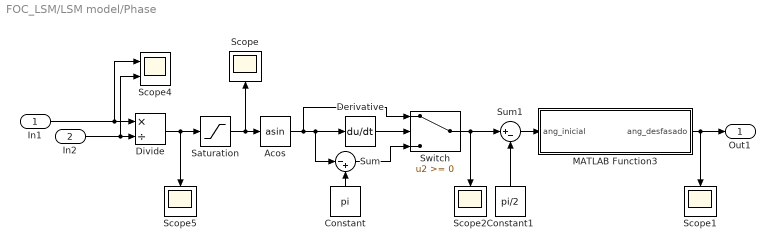
== system FOC_LSM/LSM model/Phase ==
  In1 : Inport
  In2 : Inport  Port=2
  Acos : Trigonometry  Operator=asin  OutputSignalType=real
  Constant : Constant  Value=pi
  Constant1 : Constant  Value=pi/2
  Derivative : Derivative
  Divide : Product  Inputs=*/
  MATLAB Function3 : MATLAB Function  TreatAsAtomicUnit=on
  Saturation : Saturate  UpperLimit=1  LowerLimit=-1
  Scope{,1..2,5} (4 alike) : Scope
      Scope settings: ActiveDisplayYMinimum=-1.25  ActiveDisplayYMaximum=1.25
      Scope1 settings: DataLoggingVariableName=ScopeData5
      Scope2 settings: ActiveDisplayYMinimum=-2.35619  ActiveDisplayYMaximum=5.49779  DataLoggingVariableName=ScopeData6
      Scope5 settings: ActiveDisplayYMinimum=-2.12336  ActiveDisplayYMaximum=9.10708  DataLoggingVariableName=ScopeData5
  Scope4 : Scope  NumInputPorts=2
      settings: ActiveDisplayYMinimum=32.617244020328293  ActiveDisplayYMaximum=91.889983525300607  DataLoggingVariableName=ScopeData4
  Sum : Sum  Inputs=|-+
  Sum1 : Sum  Inputs=|+-
  Switch : Switch  SaturateOnIntegerOverflow=off  InputSameDT=off
  Out1 : Outport
  wires:
  In1/1 -> Scope4/1, Divide/1
  In2/1 -> Scope4/2, Divide/2
  Divide/1 -> Scope5/1, Saturation/1
  Sum1/1 -> MATLAB Function3/1(ang_inicial)
  Constant1/1 -> Sum1/2
  Saturation/1 -> Acos/1, Scope/1
  Constant/1 -> Sum/2
  Sum/1 -> Switch/3
  Acos/1 -> Derivative/1, Sum/1, Switch/1
  Derivative/1 -> Switch/2
  Switch/1 -> Sum1/1, Scope2/1
  MATLAB Function3/1(ang_desfasado) -> Out1/1, Scope1/1

== system FOC_LSM/LSM model/Sensor de Corriente ==
  Corriente UVW : Inport
  Demux : Demux  Outputs=3
  Mux : Mux  Inputs=3
  Scope : Scope
  Sensor corriente U : Subsystem
  Sensor corriente V : Subsystem
  Sensor corriente W : Subsystem
  Corriente Medida : Outport
  wires:
  Corriente UVW/1 -> Scope/1, Demux/1
  Demux/1 -> Sensor corriente U/1(I)
  Demux/2 -> Sensor corriente V/1(I)
  Demux/3 -> Sensor corriente W/1(I)
  Mux/1 -> Corriente Medida/1
  Sensor corriente U/1(valor) -> Mux/1
  Sensor corriente W/1(valor) -> Mux/3
  Sensor corriente V/1(valor) -> Mux/2

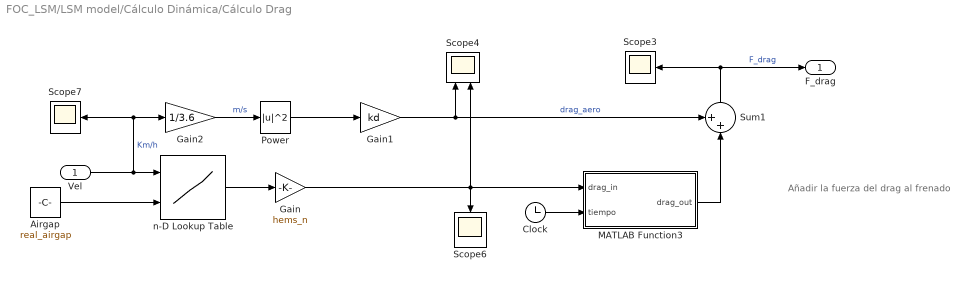
== system FOC_LSM/LSM model/Cálculo Dinámica/Cálculo Drag ==
  note: Añadir la fuerza del drag al frenado
  Vel : Inport
  Airgap : Constant  Value=real_airgap
  Clock : Clock
  Gain : Gain  Gain=hems_n
  Gain1 : Gain  Gain=kd
  Gain2 : Gain  Gain=1/3.6
  MATLAB Function3 : MATLAB Function  TreatAsAtomicUnit=on
  Power : Math  Operator=magnitude^2
  Scope3 : Scope
      settings: ActiveDisplayYMinimum=-54.120073541906933  ActiveDisplayYMaximum=99.544523919239481  DataLoggingVariableName=ScopeData17
  Scope4 : Scope  NumInputPorts=2
      settings: ActiveDisplayYMinimum=-20.482608041587291  ActiveDisplayYMaximum=116.00452047756229  DataLoggingVariableName=ScopeData18
  Scope6 : Scope
      settings: ActiveDisplayYMinimum=-41.11542  ActiveDisplayYMaximum=370.03797  DataLoggingVariableName=ScopeData19
  Scope7 : Scope
      settings: ActiveDisplayYMinimum=-6.2524  ActiveDisplayYMaximum=56.27152  DataLoggingVariableName=ScopeData20
  Sum1 : Sum  Inputs=++|
  n-D Lookup Table : Lookup_n-D  BreakpointsForDimension1=speed_drag_vec  BreakpointsForDimension2=airgap_vec  BreakpointsForDimension3=[5, 7]  Table=force_drag_vec  InternalRulePriority=Speed  RndMeth=Simplest
      settings: InputPortMap=u0,u1
  F_drag : Outport
  wires:
  Airgap/1 -> n-D Lookup Table/2
  Clock/1 -> MATLAB Function3/2(tiempo)
  Gain1/1 -> Scope4/1, Sum1/1  "drag_aero"
  Gain2/1 -> Power/1  "m/s"
  Vel/1 -> Gain2/1, Scope7/1, n-D Lookup Table/1  "Km/h"
  Sum1/1 -> F_drag/1, Scope3/1  "F_drag"
  MATLAB Function3/1(drag_out) -> Sum1/2
  Gain/1 -> MATLAB Function3/1(drag_in), Scope4/2, Scope6/1
  n-D Lookup Table/1 -> Gain/1
  Power/1 -> Gain1/1

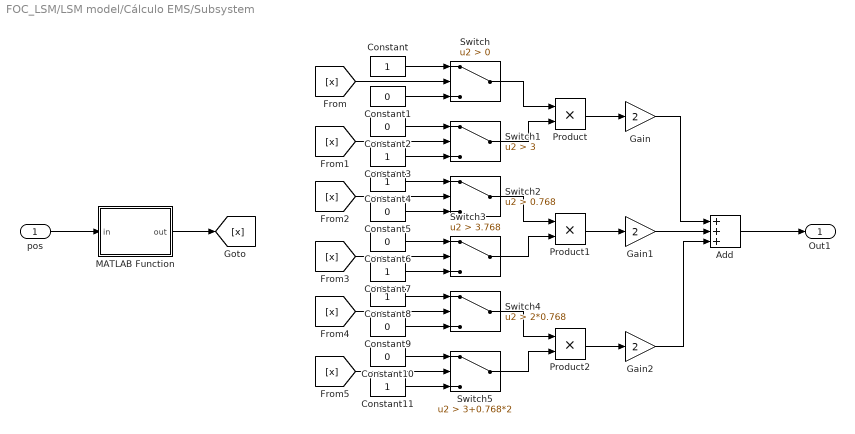
== system FOC_LSM/LSM model/Cálculo EMS/Subsystem ==
  pos : Inport
  Add : Sum  Inputs=+++
  Constant{,3..4,7..8,11} (6 alike) : Constant
  Constant{1..2,5..6,9..10} (6 alike) : Constant  Value=0
  Gain : Gain  Gain=2
  Gain1 : Gain  Gain=2
  Gain2 : Gain  Gain=2
  MATLAB Function : MATLAB Function  TreatAsAtomicUnit=on
  Product : Product
  Product1 : Product
  Product2 : Product
  Switch : Switch  Criteria=u2 > Threshold  SaturateOnIntegerOverflow=off  InputSameDT=off
  Switch1 : Switch  Criteria=u2 > Threshold  Threshold=3  SaturateOnIntegerOverflow=off  InputSameDT=off
  Switch2 : Switch  Criteria=u2 > Threshold  Threshold=0.768  SaturateOnIntegerOverflow=off  InputSameDT=off
  Switch3 : Switch  Criteria=u2 > Threshold  Threshold=3.768  SaturateOnIntegerOverflow=off  InputSameDT=off
  Switch4 : Switch  Criteria=u2 > Threshold  Threshold=2*0.768  SaturateOnIntegerOverflow=off  InputSameDT=off
  Switch5 : Switch  Criteria=u2 > Threshold  Threshold=3+0.768*2  SaturateOnIntegerOverflow=off  InputSameDT=off
  Out1 : Outport
  wires:
  pos/1 -> MATLAB Function/1(in)
  Add/1 -> Out1/1
  Product/1 -> Gain/1
  Constant1/1 -> Switch/3
  Switch/1 -> Product/1
  Product2/1 -> Gain2/1
  Gain1/1 -> Add/2
  [x] -> Switch/2
  Constant2/1 -> Switch1/1
  [x] -> Switch1/2
  Constant/1 -> Switch/1
  Switch5/1 -> Product2/2
  Switch1/1 -> Product/2
  Switch3/1 -> Product1/2
  Switch2/1 -> Product1/1
  Constant10/1 -> Switch5/1
  [x] -> Switch5/2
  Constant11/1 -> Switch5/3
  Gain/1 -> Add/1
  Product1/1 -> Gain1/1
  [x] -> Switch3/2
  Gain2/1 -> Add/3
  [x] -> Switch2/2
  Constant8/1 -> Switch4/1
  Constant6/1 -> Switch3/1
  Constant9/1 -> Switch4/3
  Constant3/1 -> Switch1/3
  Constant4/1 -> Switch2/1
  Constant7/1 -> Switch3/3
  Constant5/1 -> Switch2/3
  [x] -> Switch4/2
  Switch4/1 -> Product2/1
  MATLAB Function/1(out) -> [x]

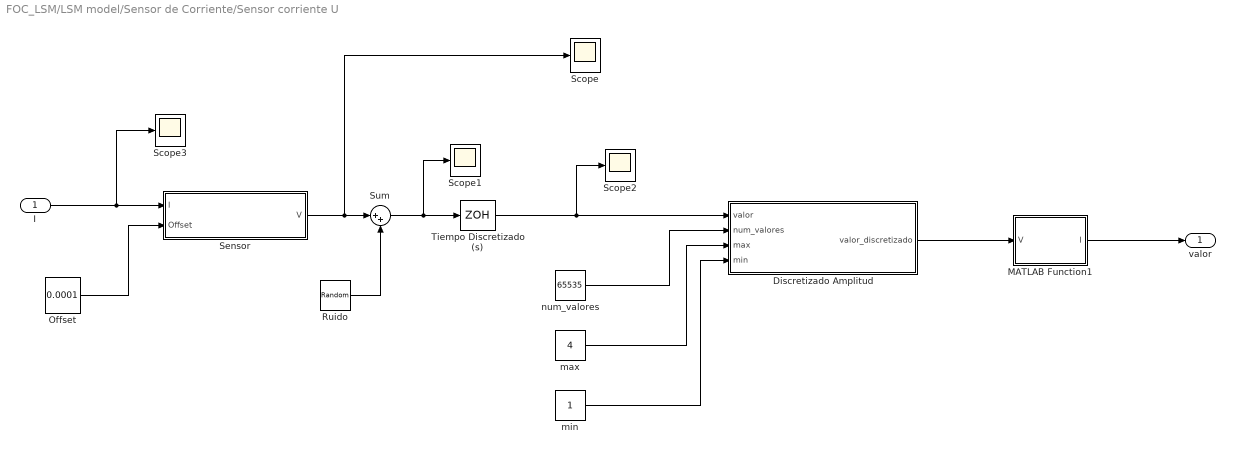
== system FOC_LSM/LSM model/Sensor de Corriente/Sensor corriente U ==
  I : Inport
  Discretizado Amplitud : MATLAB Function  TreatAsAtomicUnit=on
  MATLAB Function1 : MATLAB Function  TreatAsAtomicUnit=on
  Offset : Constant  Value=0.0001
  Ruido : RandomNumber  Variance=0.000003  Seed=10  SampleTime=0.0002
  Scope{,1..3} (4 alike) : Scope
      Scope settings: ActiveDisplayYMinimum=2.49501  ActiveDisplayYMaximum=2.50519  DataLoggingVariableName=ScopeData11
      Scope1 settings: ActiveDisplayYMinimum=2.48778  ActiveDisplayYMaximum=2.51163  DataLoggingVariableName=ScopeData12
      Scope2 settings: ActiveDisplayYMinimum=2.00149  ActiveDisplayYMaximum=2.99672  DataLoggingVariableName=ScopeData13
      Scope3 settings: ActiveDisplayYMinimum=-98.96668  ActiveDisplayYMaximum=98.65569  DataLoggingVariableName=ScopeData14
  Sensor : MATLAB Function  TreatAsAtomicUnit=on
  Sum : Sum  Inputs=|++
  Tiempo Discretizado (s) : ZeroOrderHold  SampleTime=0.0002
  max : Constant  Value=4
  min : Constant
  num_valores : Constant  Value=65535
  valor : Outport
  wires:
  I/1 -> Scope3/1, Sensor/1(I)
  Offset/1 -> Sensor/2(Offset)
  Sensor/1(V) -> Scope/1, Sum/1
  Ruido/1 -> Sum/2
  Sum/1 -> Scope1/1, Tiempo Discretizado (s)/1
  Tiempo Discretizado (s)/1 -> Scope2/1, Discretizado Amplitud/1(valor)
  num_valores/1 -> Discretizado Amplitud/2(num_valores)
  max/1 -> Discretizado Amplitud/3(max)
  min/1 -> Discretizado Amplitud/4(min)
  Discretizado Amplitud/1(valor_discretizado) -> MATLAB Function1/1(V)
  MATLAB Function1/1(I) -> valor/1

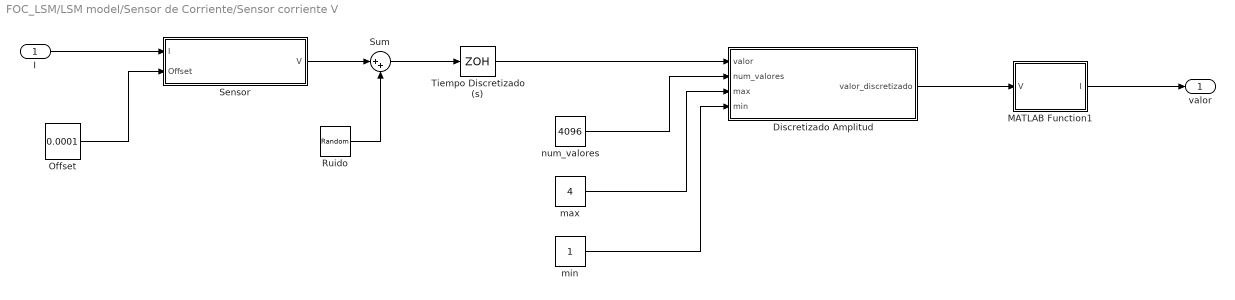
== system FOC_LSM/LSM model/Sensor de Corriente/Sensor corriente V ==
  I : Inport
  Discretizado Amplitud : MATLAB Function  TreatAsAtomicUnit=on
  MATLAB Function1 : MATLAB Function  TreatAsAtomicUnit=on
  Offset : Constant  Value=0.0001
  Ruido : RandomNumber  Variance=0.000003  Seed=10  SampleTime=0.0002
  Sensor : MATLAB Function  TreatAsAtomicUnit=on
  Sum : Sum  Inputs=|++
  Tiempo Discretizado (s) : ZeroOrderHold  SampleTime=0.0002
  max : Constant  Value=4
  min : Constant
  num_valores : Constant  Value=4096
  valor : Outport
  wires:
  MATLAB Function1/1(I) -> valor/1
  Sensor/1(V) -> Sum/1
  Offset/1 -> Sensor/2(Offset)
  min/1 -> Discretizado Amplitud/4(min)
  Tiempo Discretizado (s)/1 -> Discretizado Amplitud/1(valor)
  Ruido/1 -> Sum/2
  I/1 -> Sensor/1(I)
  Sum/1 -> Tiempo Discretizado (s)/1
  num_valores/1 -> Discretizado Amplitud/2(num_valores)
  Discretizado Amplitud/1(valor_discretizado) -> MATLAB Function1/1(V)
  max/1 -> Discretizado Amplitud/3(max)

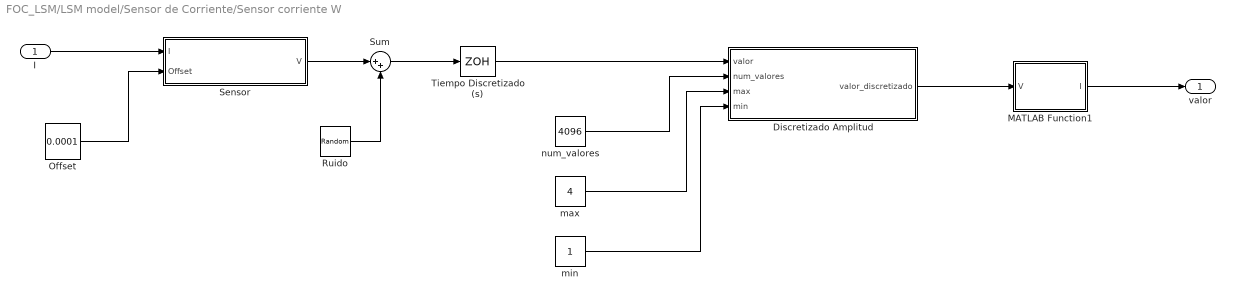
== system FOC_LSM/LSM model/Sensor de Corriente/Sensor corriente W ==
  I : Inport
  Discretizado Amplitud : MATLAB Function  TreatAsAtomicUnit=on
  MATLAB Function1 : MATLAB Function  TreatAsAtomicUnit=on
  Offset : Constant  Value=0.0001
  Ruido : RandomNumber  Variance=0.000003  Seed=10  SampleTime=0.0002
  Sensor : MATLAB Function  TreatAsAtomicUnit=on
  Sum : Sum  Inputs=|++
  Tiempo Discretizado (s) : ZeroOrderHold  SampleTime=0.0002
  max : Constant  Value=4
  min : Constant
  num_valores : Constant  Value=4096
  valor : Outport
  wires:
  MATLAB Function1/1(I) -> valor/1
  Sensor/1(V) -> Sum/1
  Offset/1 -> Sensor/2(Offset)
  min/1 -> Discretizado Amplitud/4(min)
  Tiempo Discretizado (s)/1 -> Discretizado Amplitud/1(valor)
  Ruido/1 -> Sum/2
  I/1 -> Sensor/1(I)
  Sum/1 -> Tiempo Discretizado (s)/1
  num_valores/1 -> Discretizado Amplitud/2(num_valores)
  Discretizado Amplitud/1(valor_discretizado) -> MATLAB Function1/1(V)
  max/1 -> Discretizado Amplitud/3(max)

== matlab function FOC_LSM/LSM model/Sensor de Corriente/Sensor corriente W/Discretizado Amplitud ==
  data: valor input; valor_discretizado output; num_valores input; max input; min input
function valor_discretizado = fcn(valor, num_valores, max, min)

if valor > max
    valor_discretizado = max;
    return
end

if valor < min
    valor_discretizado = min;
    return
end


valor_escalon = (max - min)/(num_valores - 1);


i = min;


while (i < max)
    if (i + valor_escalon/2 > valor)
        valor_discretizado = i;
        return
    end

    i = i + valor_escalon;
end


valor_discretizado = max;

end

== matlab function FOC_LSM/LSM model/Maximun calculation/MATLAB Function1 ==
  settings: updateMethod=DISCRETE
  data: frecuencia input; Maximo output; valor input; tiempo input
function Maximo = fcn(frecuencia,valor,tiempo)

   persistent antiguo_maximo
    if isempty(antiguo_maximo)
       antiguo_maximo=0;
    end
    persistent t_maximo
    if isempty(t_maximo)
       t_maximo=0;
    end

maximo = [0 0 0];

periodo=1/abs(frecuencia)/3;

for i=1:3
    if abs(valor(i))>=antiguo_maximo
        maximo(i)=abs(valor(i));
        antiguo_maximo=abs(valor(i));
        t_maximo=tiempo;
    else
        maximo(i)=antiguo_maximo;
        if tiempo>t_maximo+periodo
            maximo(i)=abs(valor(i));
            antiguo_maximo=abs(valor(i));
            t_maximo=tiempo;
        end
    end
end

Maximo = max(maximo);

== matlab function FOC_LSM/LSM model/Sensor de Corriente/Sensor corriente W/MATLAB Function1 ==
  data: V input; I output
function I = fcn(V)

I = (V - 2.5)/0.005;

== matlab function FOC_LSM/LSM model/Sensor de Corriente/Sensor corriente W/Sensor ==
  data: I input; V output; Offset input
function V = fcn(I, Offset)

Vcc = 5;                                        %Vcc ??                             La corriente va hasta máximo 5V

if (I > 300)
    I = 300;
end

if (I < -300)
    I = -300;
end


V_ref = Vcc / 2;

V = V_ref + 0.005 * I;

V = V + Offset;                 % Por?


end

== matlab function FOC_LSM/LSM model/Phase/MATLAB Function3 ==
  data: ang_inicial input; ang_desfasado output
function ang_desfasado = fcn(ang_inicial)


if ang_inicial < 0
    corregido = ang_inicial + 2*pi;
else
    corregido = ang_inicial;
end


desfase = corregido + 0.63;

if desfase > 2*pi
    desfase = desfase - 2*pi;
end

ang_desfasado = desfase;


end

== matlab function FOC_LSM/LSM model/Cálculo EMS/Cálculo EMS ==
  settings: updateMethod=DISCRETE
  data: laser input; pos input; numero_EMS output
function numero_EMS = fcn(laser, pos)

desfase_laser = (0.174+0.116+0.0925);
pos_EMS = pos - desfase_laser;

persistent laser_ant
if isempty(laser_ant)
    laser_ant = 0;
end

persistent pos_ref
if isempty(pos_ref)
    pos_ref = -1;
end


if laser == 1 && laser_ant == 0
    pos_ref = pos;                                % Se toma como referencia de posición el momento en que el láser detecta el booster
end



if pos_ref == -1 || pos_EMS < pos_ref || pos_EMS > pos_ref + 4.536
    numero_EMS = 0;
else
    numero_EMS = 2;

    if pos_EMS >= pos_ref + 0.768 && pos_EMS <= pos_ref + 3.768
        numero_EMS = 4;

        if pos_EMS >= pos_ref + 1.536 && pos_EMS <= pos_ref + 3
            numero_EMS = 6;
        end
    end
end


laser_ant = laser;

end

== matlab function FOC_LSM/Speetec/Speetec Detection ==
  data: pos input; speetec_detect output
function speetec_detect = fcn(pos)

if pos >= (1-0.0925) && pos <= (4+0.0925)         % Inicio y final del Booster
    speetec_detect = 1;
else
    speetec_detect = 0;
end

end

== matlab function FOC_LSM/LSM model/Cálculo EMS/Subsystem/MATLAB Function ==
  data: in input; out output
function out = fcn(in)

if in < 1
    out = 0;
else
    out = in - 1;
end

== matlab function FOC_LSM/LSM model/Cálculo Dinámica/Cálculo Drag/MATLAB Function3 ==
  data: drag_in input; drag_out output; tiempo input
function drag_out = fcn(drag_in, tiempo)

if tiempo < 1
    drag_out = 0;
else
    drag_out = drag_in;
end



%So doesn't go backward the first moment

== matlab function FOC_LSM/LSM model/Maximun calculation/MATLAB Function2 ==
  settings: updateMethod=DISCRETE
  data: frecuencia output; value input; tiempo input
function frecuencia = frecuency_calculator(value,tiempo)

   persistent signo
    if isempty(signo)
       signo=[0 0 0]; % 1 positive, 2 negative
    end
    persistent t_inicio
    if isempty(t_inicio)
       t_inicio=[0 0 0];
    end

    persistent frecuencia_acc
    if isempty(frecuencia_acc)
       frecuencia_acc=1;
    end

    frecuencia=frecuencia_acc;

    for i=1:3
    
        if signo(i) == 0
            if value(i) >= 0 
                signo(i) = 1;
            else
                signo(i) = 2;
            end
            t_inicio(i)=tiempo;
        end
        
        if signo(i)==1
            if value(i) <= 0
                frecuencia = 1/(2*(tiempo-t_inicio(i)));
                frecuencia_acc=frecuencia;
                signo(i) = 0;
            end
        end
        
        if signo(i)==2
            if value(i) >= 0
                frecuencia = 1/(2*(tiempo-t_inicio(i)));
                frecuencia_acc=frecuencia;
                signo(i) = 0;
            end
        end

    end

== matlab function FOC_LSM/Clark Park/Clarke Transform ==
  data: abc input; AlphaBeta0 output
function AlphaBeta0 = fcn(abc)

M = [1,-1/2,-1/2;0,sqrt(3)/2,-sqrt(3)/2;1/2,1/2,1/2];

AlphaBeta0 = (2/3)*(M*abc);

== matlab function FOC_LSM/Clark Park/Clarke to Park Angle Transform ==
  data: AlphaBeta0 input; dq0 output; ELE_angle input
function dq0 = fcn(AlphaBeta0, ELE_angle)

M = [sin(ELE_angle),-cos(ELE_angle),0; cos(ELE_angle),sin(ELE_angle),0; 0,0,1];

dq0 = M*AlphaBeta0;

== matlab function FOC_LSM/Reverse Park Clark/Inverse Park Transform ==
  data: dq0 input; abc output; ELE_angle input
function abc = fcn(dq0, ELE_angle)

M = [sin(ELE_angle),cos(ELE_angle),1; sin(ELE_angle-(2*pi/3)),cos(ELE_angle-(2*pi/3)),1; sin(ELE_angle+(2*pi/3)),cos(ELE_angle+(2*pi/3)),1];

abc = M*dq0;

end

== matlab function FOC_LSM/LSM model/Sensor de Corriente/Sensor corriente U/Sensor ==
  data: I input; V output; Offset input
function V = fcn(I, Offset)

Vcc = 5;                                        %Vcc ??                             La corriente va hasta máximo 5V

if (I > 300)
    I = 300;
end

if (I < -300)
    I = -300;
end


V_ref = Vcc / 2;

V = V_ref + 0.005 * I;

V = V + Offset;                 % Por?


end

== matlab function FOC_LSM/LSM model/Sensor de Corriente/Sensor corriente U/Discretizado Amplitud ==
  data: valor input; valor_discretizado output; num_valores input; max input; min input
function valor_discretizado = fcn(valor, num_valores, max, min)

if valor > max
    valor_discretizado = max;
    return
end

if valor < min
    valor_discretizado = min;
    return
end


valor_escalon = (max - min)/(num_valores - 1);


i = min;


while (i < max)
    if (i + valor_escalon/2 > valor)
        valor_discretizado = i;
        return
    end

    i = i + valor_escalon;
end


valor_discretizado = max;

end

== matlab function FOC_LSM/LSM model/Sensor de Corriente/Sensor corriente U/MATLAB Function1 ==
  data: V input; I output
function I = fcn(V)

I = (V - 2.5)/0.005;

== matlab function FOC_LSM/LSM model/Sensor de Corriente/Sensor corriente V/Discretizado Amplitud ==
  data: valor input; valor_discretizado output; num_valores input; max input; min input
function valor_discretizado = fcn(valor, num_valores, max, min)

if valor > max
    valor_discretizado = max;
    return
end

if valor < min
    valor_discretizado = min;
    return
end


valor_escalon = (max - min)/(num_valores - 1);


i = min;


while (i < max)
    if (i + valor_escalon/2 > valor)
        valor_discretizado = i;
        return
    end

    i = i + valor_escalon;
end


valor_discretizado = max;

end

== matlab function FOC_LSM/LSM model/Sensor de Corriente/Sensor corriente V/MATLAB Function1 ==
  data: V input; I output
function I = fcn(V)

I = (V - 2.5)/0.005;

== matlab function FOC_LSM/LSM model/Sensor de Corriente/Sensor corriente V/Sensor ==
  data: I input; V output; Offset input
function V = fcn(I, Offset)

Vcc = 5;                                        %Vcc ??                             La corriente va hasta máximo 5V

if (I > 300)
    I = 300;
end

if (I < -300)
    I = -300;
end


V_ref = Vcc / 2;

V = V_ref + 0.005 * I;

V = V + Offset;                 % Por?


end
